simulink model "Kalition_Test"  (R2016a)
settings: Solver=ode2  StartTime=0.0  StopTime=Tsim  FixedStep=0.01  RelTol=1e-3
values from neighbouring files (symbols this model uses):
  acc_scale = mean(acc(1:100,3))    [Kalition_test.m]
  bias_x = acc_bias(1)    [Kalition_test.m]
  bias_y = acc_bias(2)    [Kalition_test.m]
  Q = diag([q q q])    [Kalition_test.m]
  R = diag([sigma_acc^2 sigma_opti^2])    [Kalition_test.m]
  ts = 0.01    [Kalition_test.m]
settings Model: Creator=pela  LastModifiedBy=ergae
settings DataIOCC: LimitDataPoints=on  SaveFormat=Array
settings HardwareCC: ProdBitPerPointer=32  ProdLargestAtomicInteger=Long  ProdLargestAtomicFloat=Double  ProdIntDivRoundTo=Undefined  ProdWordSize=32  ProdHWDeviceType=ARM Compatible->ARM Cortex
settings ModelReferenceCC: UpdateModelReferenceTargets=Force  PropagateSignalLabelsOutOfModel=off
settings RTWCC: GenCodeOnly=on  GenerateReport=on  Toolchain=GNU gcc/g++ v4.4.x | gmake (64-bit Linux)  BuildConfiguration=Faster Runs  LaunchReport=on  TargetLang=C++
settings GRTTargetCC: MatFileLogging=off  MultiInstanceERTCode=on  CodeInterfacePackaging=C++ class  SupportNonFinite=off
settings ConfigComp: CovModelRefEnable=Off

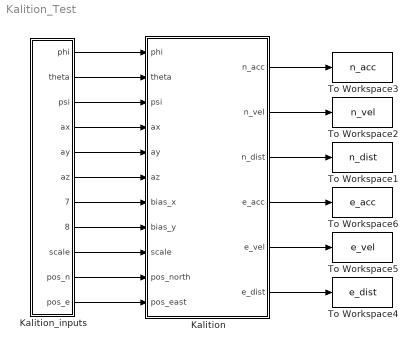
== system Kalition_Test ==
  Kalition : Subsystem
  Kalition_inputs : Subsystem
  To Workspace1 : ToWorkspace  VariableName=n_dist  SaveFormat=Timeseries  SampleTime=-1
  To Workspace2 : ToWorkspace  VariableName=n_vel  SaveFormat=Timeseries  SampleTime=-1
  To Workspace3 : ToWorkspace  VariableName=n_acc  SaveFormat=Timeseries  SampleTime=-1
  To Workspace4 : ToWorkspace  VariableName=e_dist  SaveFormat=Timeseries  SampleTime=-1
  To Workspace5 : ToWorkspace  VariableName=e_vel  SaveFormat=Timeseries  SampleTime=-1
  To Workspace6 : ToWorkspace  VariableName=e_acc  SaveFormat=Timeseries  SampleTime=-1
  wires:
  Kalition_inputs/1(phi) -> Kalition/1(phi)
  Kalition_inputs/2(theta) -> Kalition/2(theta)
  Kalition_inputs/3(psi) -> Kalition/3(psi)
  Kalition_inputs/4(ax) -> Kalition/4(ax)
  Kalition_inputs/5(ay) -> Kalition/5(ay)
  Kalition_inputs/6(az) -> Kalition/6(az)
  Kalition_inputs/9(scale) -> Kalition/9(scale)
  Kalition_inputs/10(pos_n) -> Kalition/10(pos_north)
  Kalition_inputs/11(pos_e) -> Kalition/11(pos_east)
  Kalition/2(n_vel) -> To Workspace2/1
  Kalition/1(n_acc) -> To Workspace3/1
  Kalition/6(e_dist) -> To Workspace4/1
  Kalition/5(e_vel) -> To Workspace5/1
  Kalition/4(e_acc) -> To Workspace6/1
  Kalition_inputs/7(bias_x) -> Kalition/7(bias_x)
  Kalition_inputs/8(bias_y) -> Kalition/8(bias_y)
  Kalition/3(n_dist) -> To Workspace1/1

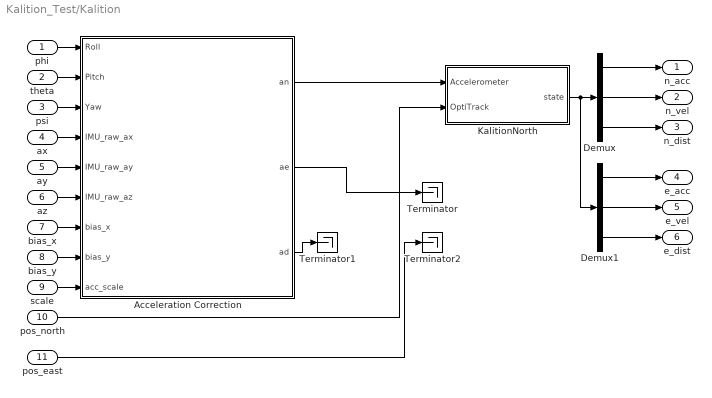
== system Kalition_Test/Kalition ==
  phi : Inport
  theta : Inport  Port=2
  psi : Inport  Port=3
  ax : Inport  Port=4
  ay : Inport  Port=5
  az : Inport  Port=6
  bias_x : Inport  Port=7
  bias_y : Inport  Port=8
  scale : Inport  Port=9
  pos_north : Inport  Port=10
  pos_east : Inport  Port=11
  Acceleration Correction : MATLAB Function  TreatAsAtomicUnit=on
  Demux : Demux  Outputs=3
  Demux1 : Demux  Outputs=3
  KalitionNorth : Subsystem
  Terminator : Terminator
  Terminator1 : Terminator
  Terminator2 : Terminator
  n_acc : Outport
  n_vel : Outport  Port=2
  n_dist : Outport  Port=3
  e_acc : Outport  Port=4
  e_vel : Outport  Port=5
  e_dist : Outport  Port=6
  wires:
  ax/1 -> Acceleration Correction/4(IMU_raw_ax)
  phi/1 -> Acceleration Correction/1(Roll)
  theta/1 -> Acceleration Correction/2(Pitch)
  ay/1 -> Acceleration Correction/5(IMU_raw_ay)
  az/1 -> Acceleration Correction/6(IMU_raw_az)
  scale/1 -> Acceleration Correction/9(acc_scale)
  Acceleration Correction/3(ad) -> Terminator1/1
  psi/1 -> Acceleration Correction/3(Yaw)
  bias_x/1 -> Acceleration Correction/7(bias_x)
  bias_y/1 -> Acceleration Correction/8(bias_y)
  Acceleration Correction/1(an) -> KalitionNorth/1(Accelerometer)
  Demux/1 -> n_acc/1
  Demux/2 -> n_vel/1
  Demux/3 -> n_dist/1
  Demux1/1 -> e_acc/1
  Demux1/2 -> e_vel/1
  Demux1/3 -> e_dist/1
  pos_north/1 -> KalitionNorth/2(OptiTrack)
  KalitionNorth/1(state) -> Demux1/1, Demux/1
  pos_east/1 -> Terminator2/1
  Acceleration Correction/2(ae) -> Terminator/1

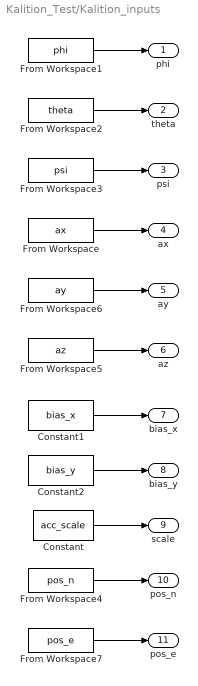
== system Kalition_Test/Kalition_inputs ==
  Constant : Constant  Value=acc_scale
  Constant1 : Constant  Value=bias_x
  Constant2 : Constant  Value=bias_y
  From Workspace : FromWorkspace  VariableName=ax  SampleTime=0
  From Workspace1 : FromWorkspace  VariableName=phi  SampleTime=0
  From Workspace2 : FromWorkspace  VariableName=theta  SampleTime=0
  From Workspace3 : FromWorkspace  VariableName=psi  SampleTime=0
  From Workspace4 : FromWorkspace  VariableName=pos_n  SampleTime=0
  From Workspace5 : FromWorkspace  VariableName=az  SampleTime=0
  From Workspace6 : FromWorkspace  VariableName=ay  SampleTime=0
  From Workspace7 : FromWorkspace  VariableName=pos_e  SampleTime=0
  phi : Outport
  theta : Outport  Port=2
  psi : Outport  Port=3
  ax : Outport  Port=4
  ay : Outport  Port=5
  az : Outport  Port=6
  bias_x : Outport  Port=7
  bias_y : Outport  Port=8
  scale : Outport  Port=9
  pos_n : Outport  Port=10
  pos_e : Outport  Port=11
  wires:
  From Workspace1/1 -> phi/1
  From Workspace2/1 -> theta/1
  From Workspace3/1 -> psi/1
  From Workspace6/1 -> ay/1
  From Workspace5/1 -> az/1
  From Workspace4/1 -> pos_n/1
  From Workspace7/1 -> pos_e/1
  Constant/1 -> scale/1
  From Workspace/1 -> ax/1
  Constant1/1 -> bias_x/1
  Constant2/1 -> bias_y/1

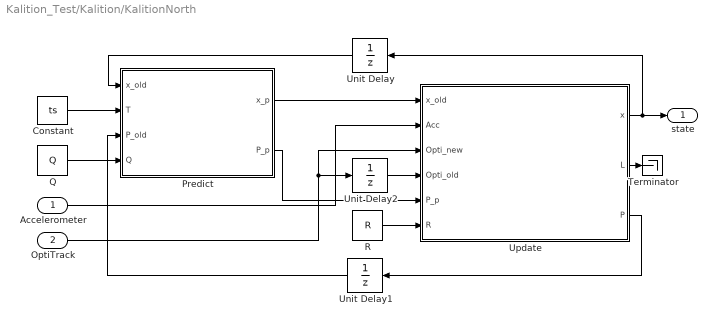
== system Kalition_Test/Kalition/KalitionNorth ==
  Accelerometer : Inport
  OptiTrack : Inport  Port=2
  Constant : Constant  Value=ts  VectorParams1D=off  SampleTime=ts
  "Predict " : MATLAB Function  TreatAsAtomicUnit=on
  Q : Constant  Value=Q  SampleTime=ts
  R : Constant  Value=R  SampleTime=ts
  Terminator : Terminator
  Unit Delay : UnitDelay  InitialCondition=zeros(3,1)  SampleTime=ts
  Unit Delay1 : UnitDelay  InitialCondition=eye(3)*0.001  SampleTime=ts
  Unit Delay2 : UnitDelay  SampleTime=ts
  Update : MATLAB Function  TreatAsAtomicUnit=on
  state : Outport
  wires:
  Unit Delay2/1 -> Update/4(Opti_old)
  OptiTrack/1 -> Update/3(Opti_new), Unit Delay2/1
  R/1 -> Update/6(R)
  Q/1 -> "Predict "/4(Q)
  Update/2(L) -> Terminator/1
  Unit Delay1/1 -> "Predict "/3(P_old)
  Update/1(x) -> Unit Delay/1, state/1
  "Predict "/1(x_p) -> Update/1(x_old)
  Accelerometer/1 -> Update/2(Acc)
  "Predict "/2(P_p) -> Update/5(P_p)
  Constant/1 -> "Predict "/2(T)
  Update/3(P) -> Unit Delay1/1
  Unit Delay/1 -> "Predict "/1(x_old)

== matlab function Kalition_Test/Kalition/Acceleration Correction ==
  data: an output; ae output; ad output; Roll input; Pitch input; Yaw input; IMU_raw_ax input; IMU_raw_ay input; IMU_raw_az input; bias_x input; bias_y input; acc_scale input
function [an,ae,ad] = Accelerometer_correction(Roll,Pitch,Yaw,IMU_raw_ax,IMU_raw_ay,IMU_raw_az,bias_x,bias_y,acc_scale)
%#codegen
% acc = [10 10 10];
acc = [IMU_raw_ax IMU_raw_ay IMU_raw_az];
%% Rotate IMU frame to the body frame
phi = pi;
theta = 0;
psi = pi/2;

Sphi = sin(phi);
Cphi = cos(phi);
Stheta = sin(theta);
Ctheta = cos(theta);
Spsi = sin(psi);
Cpsi = cos(psi);


Rx = [1   0    0   ;
      0  Cphi Sphi ;
      0 -Sphi Cphi];
Ry = [Ctheta 0 -Stheta ;
        0    1    0    ;
      Stheta 0  Ctheta];
Rz = [ Cpsi Spsi 0 ;
      -Spsi Cpsi 0 ;
        0    0   1];

acc = acc - ones(size(acc))*diag([bias_x bias_y 0]);

Acc_IMU = acc'./acc_scale;

Acc_body = Rx*Ry*Rz * Acc_IMU;
Acc_body = Acc_body' * 9.81;

%% Rotate Acc_body to Earth frame
% Roll=0.1;
% Pitch=0.1;
% Yaw= 0.1;

phi = Roll*pi/180;
theta = Pitch*pi/180;
psi = Yaw*pi/180;

Sphi = sin(phi);
Cphi = cos(phi);
Stheta = sin(theta);
Ctheta = cos(theta);
Spsi = sin(psi);
Cpsi = cos(psi);

AccEarth = zeros(size(Acc_body));
    Rx = [1     0       0    ;
          0  Cphi  Sphi ;
          0 -Sphi  Cphi];
    Ry = [Ctheta  0 -Stheta  ;
             0      1      0     ;
          Stheta  0  Ctheta ];
    Rz = [ Cpsi   Spsi   0 ;
          -Spsi  Cpsi   0 ;
              0       0    1];
    Tbet = (Rx*Ry*Rz)';
    
    accearth = Tbet * Acc_body';
    AccEarth = accearth' + [0 0 9.81];
    
an=AccEarth(1);
ae=AccEarth(2);
ad=AccEarth(3);

== matlab function Kalition_Test/Kalition/KalitionNorth/Predict  ==
  data x_old settings: description=State estimate at the previous step.
  data x_p settings: description=A-priori state estimate.
  data T settings: description=Control signal at the previous step.
  data P_p settings: description=A-priori covariance estimate.
  data P_old settings: description=Covariance estimate at the previous step.
  data: x_old input; x_p output; T input; P_p output; P_old input; Q input
%%%%%%%%%%%%%%%%%%%%%%%%%%%%%
% Kalman Position - Predict %
% Author: A.Sorbelli        %
% Date: 16/05/30            %
%%%%%%%%%%%%%%%%%%%%%%%%%%%%%

function [x_p,P_p] = state_predict(x_old,T,P_old,Q)
%% Dynamics matrix
A = [ 1 T T^2/2 ;
      0 1   T   ;
      0 0   1  ];

x_p = A*x_old;

%% Covariance propagation
P_p = A*P_old*A' + Q;

== matlab function Kalition_Test/Kalition/KalitionNorth/Update ==
  data x_old settings: description=A-priori state estimate.
  data Acc settings: description=Measurements from the sensors.
  data x settings: description=Corrected state estimate.
  data P_p settings: description=A-priori covariance estimate.
  data P settings: description=Corrected covariance estimate.
  data: x_old input; Acc input; Opti_new input; Opti_old input; x output; L output; P_p input; P output; R input
%%%%%%%%%%%%%%%%%%%%%%%%%%%%%
% Kalman Position - Update  %
% Author: A.Sorbelli        %
% Date: 16/05/30            %
%%%%%%%%%%%%%%%%%%%%%%%%%%%%%

function [x,L,P] = state_update(x_old,Acc,Opti_new,Opti_old,P_p,R)
C = [1 0 0 ;
     0 0 1];

%%
y_est = C*x_old;

%%
Pk = P_p;
x_p = x_old;

%% Accelerometer
% Innovation covariance
S = C(1,:) * Pk * C(1,:)' + R(1,1);

% Kalman gain
L = Pk*C(1,:)'/S;

% Updated state estimate
x_p = x_p + L*(Acc - y_est(1,1));

% Updated estimated covariance
Pk = (eye(3) - L*C(1,:))*Pk*(eye(3) - L*C(1,:))' + L*R(1,1)*L';

%% Optitrack
% Innovation covariance
S = C(2,:) * Pk * C(2,:)' + R(2,2);

% Kalman gain
L = Pk*C(2,:)'/S;

% Updated state estimate
x_p = x_p + L*(Opti_new - y_est(2,1));

% Updated estimated covariance
Pk = (eye(3) - L*C(2,:))*Pk*(eye(3) - L*C(2,:))' + L*R(2,2)*L';

P = Pk;
x = x_p;
